simulink model "slcenter"  (R2024a)
settings: Solver=VariableStepAuto  StartTime=0.0  StopTime=10.0  RelTol=1e-3
undefined symbols (not defined in the file or in its folder): ft, m, s
libraries: rfports1 x1, aerolibconvert2 x1, neural x1
settings Model: Creator=marisao  LastModifiedBy=marisao

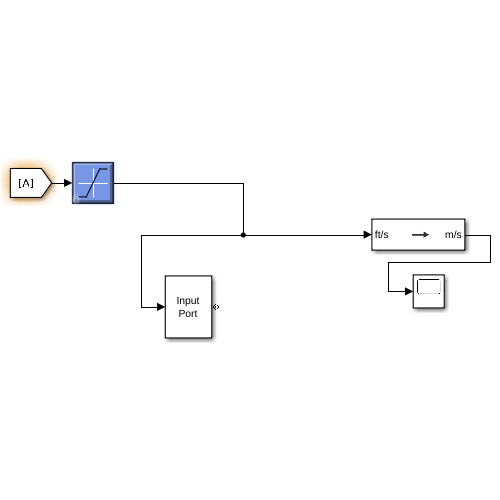
[thumbnail: Simulink's stored preview of the top-level diagram]
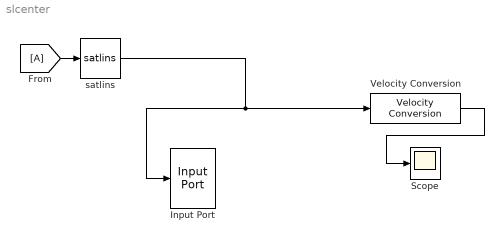
== system slcenter ==
  From : From
  Input Port : rfports1/Input Port  Description=source block  TreatSimulinkInputSignalAs=Source voltage  MaxLength=128  FracBW=0  ModelDelay=0  Fc=2e9  Ts=1e-7  Zs=50  RFhasDSP=Elements as channels (sample based)  NoiseFlag=on  seed=67987  GoToTag=RFTag
  Scope : Scope
  Velocity Conversion : aerolibconvert2/Velocity Conversion  IU=ft/s  OU=m/s
  satlins : neural/Transfer Functions/satlins
  wires:
  satlins/1 -> Input Port/1, Velocity Conversion/1
  Velocity Conversion/1 -> Scope/1
  From/1 -> satlins/1
